simulink model "Pure_Pursuit_Simulation"  (R2022b)
settings: Solver=VariableStepAuto  StartTime=0.0  StopTime=inf  RelTol=1e-3
values from neighbouring files (symbols this model uses):
  D = 3    [dataVisualizer.m]    (also in tunningPP.m)
  xRef = xRef2s    [dataVisualizer.m]    (also in tunningPP.m)
  yRef = yRef2s    [dataVisualizer.m]    (also in tunningPP.m)
undefined symbols (not defined in the file or in its folder): esc, hz, L, ld, path
libraries: vehdynlibviscommon x1, dspstat3 x1, autolibshared x1
settings Model: Creator=kisho  LastModifiedBy=kisho
settings DebuggingCC: UnconnectedInputMsg=warning  UnconnectedOutputMsg=warning  UnconnectedLineMsg=warning
settings ModelReferenceCC: EnableRefExpFcnMdlSchedulingChecks=on
settings RTWCC: DLArmComputeVersion=19.05

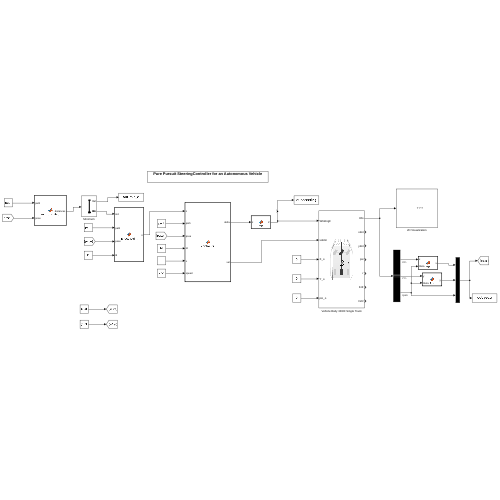
[thumbnail: Simulink's stored preview of the top-level diagram]
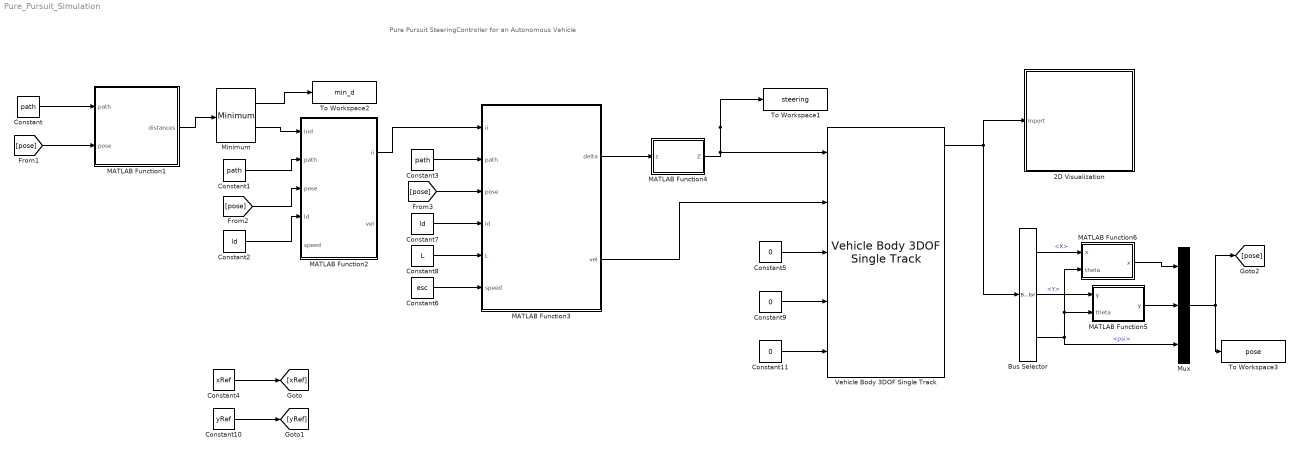
== system Pure_Pursuit_Simulation ==
  note: Pure Pursuit SteeringController for an Autonomous Vehicle
  2D Visualization : Subsystem
      mask Display: image("visualization.JPG");
  Bus Selector : BusSelector  OutputSignals=InertFrm.Cg.Disp.X,InertFrm.Cg.Disp.Y,InertFrm.Cg.Ang.psi
  Constant : Constant  Value=path  SampleTime=1/hz
  Constant1 : Constant  Value=path  SampleTime=1/hz
  Constant10 : Constant  Value=yRef  SampleTime=1/hz
  Constant11 : Constant  Value=0  SampleTime=1/hz
  Constant2 : Constant  Value=ld  SampleTime=1/hz
  Constant3 : Constant  Value=path  SampleTime=1/hz
  Constant4 : Constant  Value=xRef  SampleTime=1/hz
  Constant5 : Constant  Value=0  SampleTime=1/hz
  Constant6 : Constant  Value=esc  SampleTime=1/hz
  Constant7 : Constant  Value=ld  SampleTime=1/hz
  Constant8 : Constant  Value=L  SampleTime=1/hz
  Constant9 : Constant  Value=0  SampleTime=1/hz
  MATLAB Function1 : MATLAB Function  TreatAsAtomicUnit=on
  MATLAB Function2 : MATLAB Function  TreatAsAtomicUnit=on
  MATLAB Function3 : MATLAB Function  TreatAsAtomicUnit=on
  MATLAB Function4 : MATLAB Function  TreatAsAtomicUnit=on
  MATLAB Function5 : MATLAB Function  TreatAsAtomicUnit=on
  MATLAB Function6 : MATLAB Function  TreatAsAtomicUnit=on
  Minimum : dspstat3/Minimum  operation=minimum  fcn=Value and Index  indexBase=One  operateOver=Each row  Dimension=1  InputProcessing=Columns as channels (frame based)  reset=None  roiEnable=off  roiType=Rectangles  roiPortion=Entire ROI  roiOutput=Individual statistics for each ROI  roiFlag=off  roundingMode=Floor  overflowMode=off
      settings: LibrarySourceBlock=dsphdlsupportstat/Minimum
  Mux : Mux  Inputs=3
  To Workspace1 : ToWorkspace  VariableName=steering  SaveFormat=Structure With Time  SampleTime=1/hz
  To Workspace2 : ToWorkspace  VariableName=min_d  SaveFormat=Structure With Time  SampleTime=-1
  To Workspace3 : ToWorkspace  VariableName=pose  SaveFormat=Structure With Time  SampleTime=-1
  Vehicle Body 3DOF Single Track : autolibshared/Vehicle Body 3DOF Single Track  trackMode=Single (bicycle)  inputMode=External longitudinal velocity  frontSteerMode=on  rearSteerMode=off  windMode=off  muMode=off  extFMode=off  extMMode=off  htchFMode=off  htchMMode=off  extXo=on  extpsio=on  extxdoto=off  extro=off  extYo=on  extTamb=off  extydoto=off  aMode=2  NF=2  NR=2  m=5  a=0.15  b=0.15  h=0  dh=1  hh=0.2  X_o=0  xdot_o=0  CalphaMode=off  sigmaMode=on  d=0  hl=0  w=[1.4,1.4]  Cy_f=12e3  Cy_r=11e3  sigma_f=.1  sigma_r=.1  alpha_f_brk=[-.1 .1]  Cy_f_data=[-9e3 9e3]  alpha_r_brk=[-.1 .1]  Cy_r_data=[-9e3 9e3]  Y_o=0  ydot_o=0  Izz=0.05  psi_o=0  r_o=0  Af=2  Cd=.3  Cl=.1  Cpm=.1  beta_w=[0 0.01:0.01:0.3]  Cs=[0 0.01:0.01:0.3]  Cym=[0 1e-6:0.01:0.3]  Pabs=101325  Tair=273  g=9.81  mu=1  xdot_tol=.01  Fznom=5000  Fxtire_sat=7e4  Fytire_sat=7e4  longOff=0  latOff=0  vertOff=0  wrapAng=off
  wires:
  MATLAB Function3/1(delta) -> MATLAB Function4/1(z)
  MATLAB Function2/1(ii) -> MATLAB Function3/1(ii)
  Constant7/1 -> MATLAB Function3/4(ld)
  Constant1/1 -> MATLAB Function2/2(path)
  Constant3/1 -> MATLAB Function3/2(path)
  [pose] -> MATLAB Function3/3(pose)
  [pose] -> MATLAB Function2/3(pose)
  MATLAB Function1/1(distances) -> Minimum/1
  Minimum/2 -> MATLAB Function2/1(ind)
  Constant2/1 -> MATLAB Function2/4(ld)
  [pose] -> MATLAB Function1/2(pose)
  Constant/1 -> MATLAB Function1/1(path)
  Constant8/1 -> MATLAB Function3/5(L)
  Constant6/1 -> MATLAB Function3/6(speed)
  Constant4/1 -> [xRef]
  Constant10/1 -> [yRef]
  Bus Selector/2 -> MATLAB Function5/1("y ")  "<Y>"
  Mux/1 -> [pose], To Workspace3/1
  MATLAB Function6/1(x) -> Mux/1
  Constant5/1 -> Vehicle Body 3DOF Single Track/3
  Bus Selector/1 -> MATLAB Function6/1("x ")  "<X>"
  Constant9/1 -> Vehicle Body 3DOF Single Track/4
  Constant11/1 -> Vehicle Body 3DOF Single Track/5
  MATLAB Function4/1(Z) -> Vehicle Body 3DOF Single Track/1, To Workspace1/1
  Vehicle Body 3DOF Single Track/1 -> Bus Selector/1, 2D Visualization/1(Inport)
  Bus Selector/3 -> Mux/3, MATLAB Function5/2(theta), MATLAB Function6/2(theta)  "<psi>"
  MATLAB Function5/1(y) -> Mux/2
  MATLAB Function3/2(vel) -> Vehicle Body 3DOF Single Track/2
  Minimum/1 -> To Workspace2/1

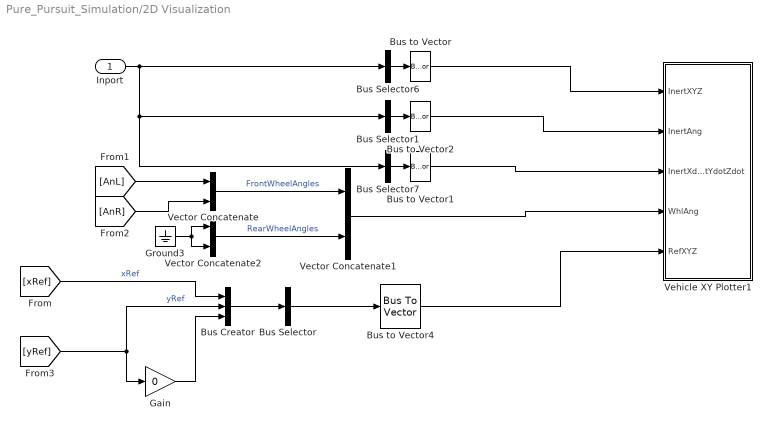
== system Pure_Pursuit_Simulation/2D Visualization ==
  Inport : Inport
  Bus Creator : BusCreator  Inputs=3
  Bus Selector : BusSelector  OutputSignals=xRef,yRef,signal3  OutputAsBus=on
  Bus Selector1 : BusSelector  OutputSignals=InertFrm.Cg.Ang.phi,InertFrm.Cg.Ang.theta,InertFrm.Cg.Ang.psi  OutputAsBus=on
  Bus Selector6 : BusSelector  OutputSignals=InertFrm.Geom.Disp.X,InertFrm.Geom.Disp.Y,InertFrm.Geom.Disp.Z  OutputAsBus=on
  Bus Selector7 : BusSelector  OutputSignals=InertFrm.Geom.Vel.Xdot,InertFrm.Geom.Vel.Ydot,InertFrm.Geom.Vel.Zdot  OutputAsBus=on
  Bus to Vector{,1..2,4} (4 alike) : BusToVector
  Gain : Gain  Gain=0
  Ground3 : Ground
  Vector Concatenate : Concatenate
  Vector Concatenate1 : Concatenate
  Vector Concatenate2 : Concatenate
  Vehicle XY Plotter1 : Subsystem  mask(Vehicle XY Plotter){extRef=on, extStats=off, extTireF=off, a=2, b=2, w=2, figBorder=10, bufferSize=1024, velNorm=5, tireFNorm=1000, pltDT=0.2}
      mask prompts: extRef "Plot path reference, extRef"; extStats "Display speed, RPM and Gear"; extTireF "Display tire forces"; a "Distance to front axle from CG, a [m]:"; b "Distance to rear axle from CG, b [m]:"; w "Track width, w [m]:"; figBorder "Distance to figure borders, figBorder [m]:"; bufferSize "Path buffer sampe size, bufferSize []:"; velNorm "Velocity vector scaling, velNorm [m*s/m]:"; tireFNorm "Tire force vector scaling, tireFNorm [m/N]:"; pltDT "Plot update rate, pltDT [s]:"
      mask help:
      | This block will display a MATLAB figure which indicates the vehicle path, current position and heading velocity.
      | An optional path reference is also provided.
      mask init:
      | block = gcb;
      | if autoblkschecksimstopped(block)
      |     ParamNames = {'extRef';'extStats';'extTireF';'extTireF'};
      |     PortNames = {'RefXYZ';'Stats';'TireFx';'TireFy'};
      |     for idx=1:length(PortNames)
      |         InportOption  = {'built-in/Ground', [PortNames{idx}, ' Ground'];...
      |             'built-in/Inport',PortNames{idx}};
      |         if ~strcmp(get_param(block,ParamNames{idx}),'on')
      |             NewBlkHdl = autoblksreplaceblock(block, InportOption, 1);
      |             set_param(NewBlkHdl, 'ShowName', 'off');
      |         else
      |             autoblksreplaceblock(block, InportOption, 2);
      |         end
      |     end
      |     InportNames = {'InertXYZ';'InertAng';'InertXdotYdotZdot';'WhlAng';'RefXYZ';'Stats';'TireFx';'TireFy'};
      |     FoundNames = get_param(find_system(block, 'LookUnderMasks', 'all', 'SearchDepth', 1, 'FollowLinks', 'on', 'BlockType', 'Inport'), 'Name');
      |     [~,PortI] = intersect(InportNames, FoundNames);
      |     PortI = sort(PortI);
      |     for idx = 1:length(PortI)
      |         set_param([block, '/', InportNames{PortI(idx)}], 'Port', num2str(idx));
      |     end
      | end
      mask TypeOptions a: Vehicle XY Plotter/a
      mask TypeOptions b: Vehicle XY Plotter/b
      mask TypeOptions w: Vehicle XY Plotter/w
      mask TypeOptions figBorder: Vehicle XY Plotter/figBorder
      mask TypeOptions bufferSize: Vehicle XY Plotter/bufferSize
      mask TypeOptions velNorm: Vehicle XY Plotter/velNorm
      mask TypeOptions tireFNorm: Vehicle XY Plotter/tireFNorm
      mask DialogControl Container3 Prompt: Plot and Display Options
  wires:
  Bus Creator/1 -> Bus Selector/1
  [xRef] -> Bus Creator/1  "xRef"
  Gain/1 -> Bus Creator/3
  [yRef] -> Gain/1, Bus Creator/2  "yRef"
  Bus Selector/1 -> Bus to Vector4/1
  Bus to Vector4/1 -> Vehicle XY Plotter1/5(RefXYZ)
  Inport/1 -> Bus Selector6/1, Bus Selector1/1, Bus Selector7/1
  [AnR] -> Vector Concatenate/2
  Bus Selector1/1 -> Bus to Vector2/1
  Bus to Vector2/1 -> Vehicle XY Plotter1/2(InertAng)
  Bus to Vector/1 -> Vehicle XY Plotter1/1(InertXYZ)
  Bus to Vector1/1 -> Vehicle XY Plotter1/3(InertXdotYdotZdot)
  Bus Selector7/1 -> Bus to Vector1/1
  Vector Concatenate2/1 -> Vector Concatenate1/2  "RearWheelAngles"
  [AnL] -> Vector Concatenate/1
  Vector Concatenate/1 -> Vector Concatenate1/1  "FrontWheelAngles"
  Bus Selector6/1 -> Bus to Vector/1
  Ground3/1 -> Vector Concatenate2/2, Vector Concatenate2/1
  Vector Concatenate1/1 -> Vehicle XY Plotter1/4(WhlAng)

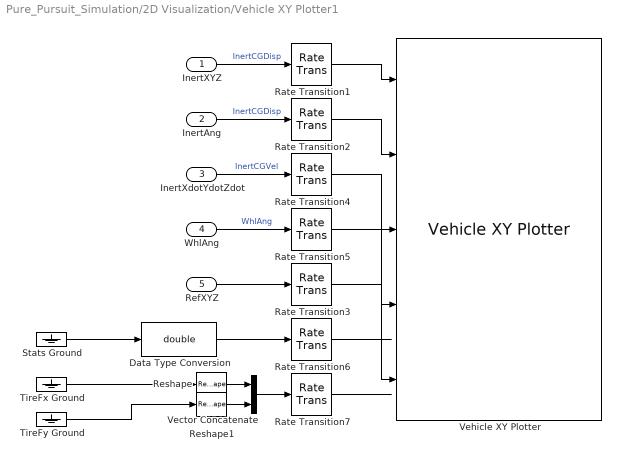
== system Pure_Pursuit_Simulation/2D Visualization/Vehicle XY Plotter1 ==
  InertXYZ : Inport
  InertAng : Inport  Port=2
  InertXdotYdotZdot : Inport  Port=3
  WhlAng : Inport  Port=4
  RefXYZ : Inport  Port=5
  Data Type Conversion : DataTypeConversion  OutDataTypeStr=double  SaturateOnIntegerOverflow=off  RndMeth=Floor
  Rate Transition{1..7} (7 alike) : RateTransition  Deterministic=off  OutPortSampleTime=pltDT
  Reshape : Reshape  OutputDimensionality=Row vector (2-D)
  Reshape1 : Reshape  OutputDimensionality=Row vector (2-D)
  Stats Ground : Ground
  TireFx Ground : Ground
  TireFy Ground : Ground
  Vector Concatenate : Concatenate  Mode=Multidimensional array
  Vehicle XY Plotter : vehdynlibviscommon/Vehicle XY Plotter  w=w  a=a  b=b  figBorder=figBorder  bufferSize=bufferSize  extStats=off  extTireF=off
  wires:
  TireFy Ground/1 -> Reshape1/1
  TireFx Ground/1 -> Reshape/1
  Stats Ground/1 -> Data Type Conversion/1
  InertAng/1 -> Rate Transition2/1  "InertCGDisp"
  InertXdotYdotZdot/1 -> Rate Transition4/1  "InertCGVel"
  InertXYZ/1 -> Rate Transition1/1  "InertCGDisp"
  WhlAng/1 -> Rate Transition5/1  "WhlAng"
  Rate Transition3/1 -> Vehicle XY Plotter/5
  Rate Transition1/1 -> Vehicle XY Plotter/1
  Rate Transition2/1 -> Vehicle XY Plotter/2
  Rate Transition4/1 -> Vehicle XY Plotter/3
  Rate Transition5/1 -> Vehicle XY Plotter/4
  Rate Transition6/1 -> ?
  Data Type Conversion/1 -> Rate Transition6/1
  Rate Transition7/1 -> ?
  RefXYZ/1 -> Rate Transition3/1
  Reshape/1 -> Vector Concatenate/1
  Reshape1/1 -> Vector Concatenate/2
  Vector Concatenate/1 -> Rate Transition7/1

== matlab function Pure_Pursuit_Simulation/MATLAB Function1 ==
  data: path input; distances output; pose input
function distances  = min_dist_find(path,pose)
 s = length(path);
 dx = zeros(1,s);
 dy = zeros(1,s);
 d  = zeros(1,s);
 for i = 1:s
     dx(i) = path(i,1) - pose(1);
     dy(i) = path(i,2) - pose(2);
 end
 distances = sqrt(dx.^2 + dy.^2);
end

== matlab function Pure_Pursuit_Simulation/MATLAB Function5 ==
  data: y input; y output; theta input
function y = fcn(y,theta)

y = y + 0.15*sin(theta);
end

== matlab function Pure_Pursuit_Simulation/MATLAB Function2 ==
  data: ind input; ii output; path input; pose input; ld input; speed input; vel output
% function ii = Target_point(ind,path,pose,ld)
% ii = ind + 1;
% 
% dist = sqrt((path(ii,1)-pose(1))^2 + (path(ii,2)-pose(2))^2);
% 
% while (dist<ld)
%     ii = ii + 1;
%     dist = sqrt((path(ii,1)-pose(1))^2 + (path(ii,2)-pose(2))^2);
% end
% 
% end



%%%%%%%%%%%%%%%%%%%%%%%%%%%%%%%%%%%%%%%%%
function [ii,vel] = Target_point(ind,path,pose,ld,speed)
ii = ind + 1;

dist = sqrt((path(ii,1)-pose(1))^2 + (path(ii,2)-pose(2))^2);
vel = speed;
while (dist<ld)
    ii = ii + 1;
    if ii >= length(path)
        vel = 0;
    else
        vel = speed;
    end


    dist = sqrt((path(ii,1)-pose(1))^2 + (path(ii,2)-pose(2))^2);
end

end

== matlab function Pure_Pursuit_Simulation/MATLAB Function3 ==
  data: delta output; vel output; ii input; path input; pose input; ld input; L input; speed input
function [delta,vel] = controller(ii,path,pose,ld,L,speed)

%%%%%%%%%%%%%%%%%%%%%%%%%%%%%%%%%%%%%%%%%%%%

% dx = path(ii,1)- pose(1);
% dy = path(ii,2)- pose(2);
% angle = atan2(dy,dx);
% if(angle < 0)
%     angle = pi + (pi +angle);
% else
% end
% alpha = (angle - pose(3));
% k = 2*sin(alpha)/ld;
% delta = atan(k*L);

%%%%%%%%%%%%%%%%%%%%%%%%%%%%%%%%%%%%%%%%%%%%

dx = path(ii,1)- pose(1);
dy = path(ii,2)- pose(2);
angle = atan2(dy,dx);
if(angle < 0)
    angle = pi + (pi +angle);
else
end
alpha = (angle - pose(3));

if alpha <= -pi
    alpha = angle + (2*pi-pose(3));
elseif alpha >= pi
    alpha = -(2*pi-angle+pose(3));
end


k = 2*sin(alpha)/ld;
delta = atan(k*L);

%%%%%%%%%%%%%%%%%%%%%%%%%%%%%%%%%%%%%%%%%%%%%
if (ii>length(path))
    vel = 0;
    delta = 0;
   
else
    vel=speed;


end

== matlab function Pure_Pursuit_Simulation/MATLAB Function4 ==
  data: z input; Z output
function Z = fcn(z)

if (z > pi/6)
    z = pi/6;
elseif (z < -pi/6)
    z = -pi/6;
else
    z =z;
end

Z = z;
end

== matlab function Pure_Pursuit_Simulation/MATLAB Function6 ==
  data: x input; x output; theta input
function x = fcn(x,theta)

x = x + 0.15*cos(theta);
end
